simulink model "Hodgkin_Huxley"  (R2019a)
settings: Solver=VariableStepAuto  StartTime=0.0  StopTime=50  RelTol=1e-9
values from neighbouring files (symbols this model uses):
  C = 1    [H_H.m]    (also in H_H_Mod.m)
  E_k = -12    [H_H.m]    (also in H_H_Mod.m)
  E_L = 10.613    [H_H.m]    (also in H_H_Mod.m)
  E_na = 115    [H_H.m]    (also in H_H_Mod.m)
  G_k = 36    [H_H.m]    (also in H_H_Mod.m)
  G_L = 0.3    [H_H.m]    (also in H_H_Mod.m)
  G_na = 120    [H_H.m]    (also in H_H_Mod.m)
  H_init = .596    (= 0.596)    [H_H.m]    (also in H_H_Mod.m)
  I_stim = 10    [H_H.m]    (also in H_H_Mod.m = 5)
  M_init = 5.296E-2    (= 0.05296)    [H_H.m]    (also in H_H_Mod.m)
  m_pow = 5    [H_H.m]    (also in H_H_Mod.m = 3)
  N_init = 0.3177    [H_H.m]    (also in H_H_Mod.m)
  n_pow = 4    [H_H.m]    (also in H_H_Mod.m)
  t_n_gain = 3    [H_H.m]    (also in H_H_Mod.m = 1)
  T_stim_start = 10    [H_H.m]    (also in H_H_Mod.m = 1)
  T_stim_stop = 15    [H_H.m]    (also in H_H_Mod.m = 5)
  V_init = 0    [H_H.m]    (also in H_H_Mod.m)
settings Model: Creator=Pranav Maddula  LastModifiedBy=Pranav Maddula

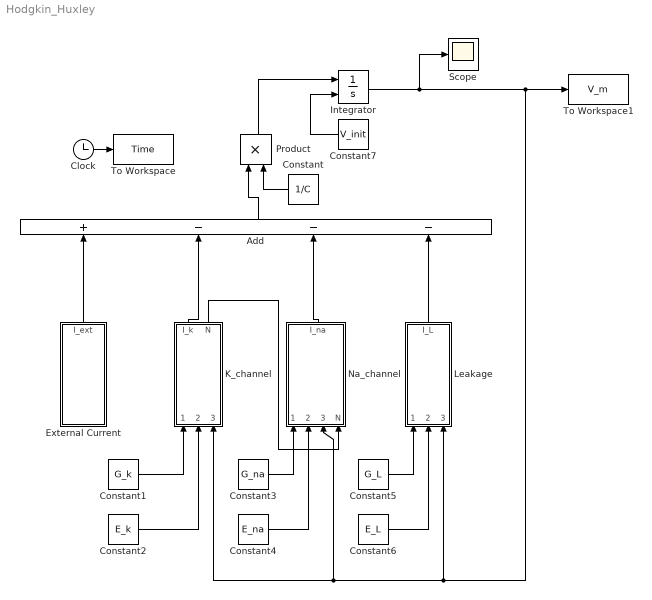
== system Hodgkin_Huxley ==
  Add : Sum  Inputs=+---
  Clock : Clock
  Constant : Constant  Value=1/C
  Constant1 : Constant  Value=G_k
  Constant2 : Constant  Value=E_k
  Constant3 : Constant  Value=G_na
  Constant4 : Constant  Value=E_na
  Constant5 : Constant  Value=G_L
  Constant6 : Constant  Value=E_L
  Constant7 : Constant  Value=V_init
  External Current : Subsystem
  Integrator : Integrator  InitialConditionSource=external
  K_channel : Subsystem
  Leakage : Subsystem
  Na_channel : Subsystem
  Product : Product
  Scope : Scope
  To Workspace : ToWorkspace  VariableName=Time  SampleTime=-1
  To Workspace1 : ToWorkspace  VariableName=V_m  SampleTime=-1
  wires:
  Clock/1 -> To Workspace/1
  External Current/1(I_ext) -> Add/1
  Leakage/1(I_L) -> Add/4
  Add/1 -> Product/1
  Constant/1 -> Product/2
  Product/1 -> Integrator/1
  Integrator/1 -> To Workspace1/1, K_channel/3(V_m), Na_channel/3(V_m), Leakage/3(V_m), Scope/1
  Constant5/1 -> Leakage/1(G_L)
  Constant6/1 -> Leakage/2(E_L)
  Constant7/1 -> Integrator/2
  K_channel/1(I_k) -> Add/2
  Na_channel/1(I_na) -> Add/3
  Constant1/1 -> K_channel/1(G_k)
  Constant2/1 -> K_channel/2(E_k)
  Constant3/1 -> Na_channel/1(G_na)
  Constant4/1 -> Na_channel/2(E_na)
  K_channel/2("N ") -> Na_channel/4(N)

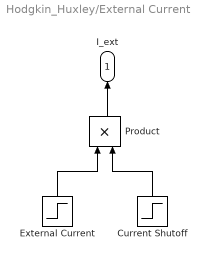
== system Hodgkin_Huxley/External Current ==
  Current Shutoff : Step  Time=T_stim_stop  Before=1  After=0  SampleTime=0
  External Current : Step  Time=T_stim_start  After=I_stim  SampleTime=0
  Product : Product
  I_ext : Outport
  wires:
  Product/1 -> I_ext/1
  External Current/1 -> Product/1
  Current Shutoff/1 -> Product/2

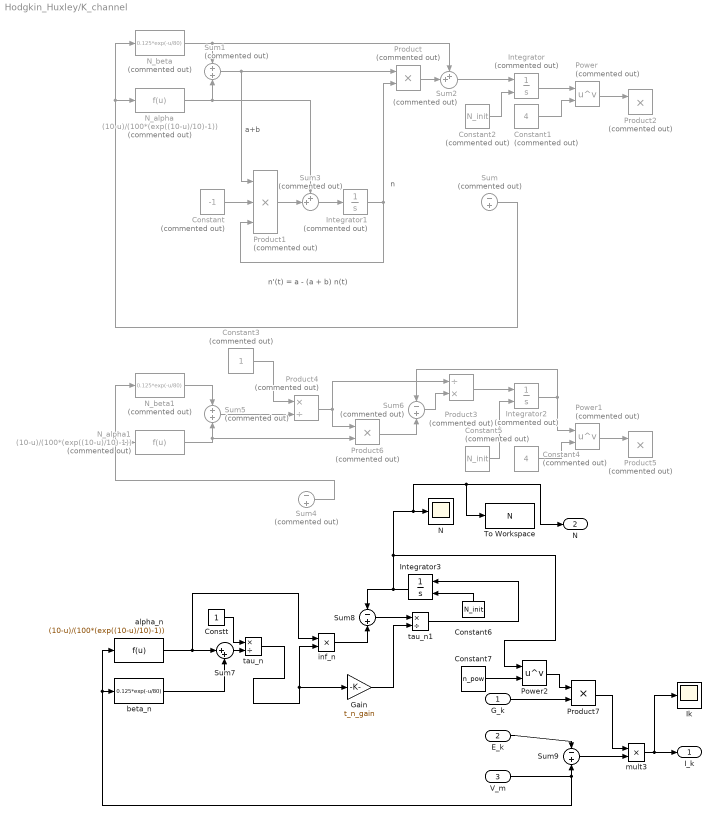
== system Hodgkin_Huxley/K_channel ==
  note: a+b
  note: n
  note: n'(t) = a - (a + b) n(t)
  G_k : Inport
  E_k : Inport  Port=2
  V_m : Inport  Port=3
  Constant : Constant  Commented=on  Value=-1
  Constant1 : Constant  Commented=on  Value=4
  Constant2 : Constant  Commented=on  Value=N_init
  Constant3 : Constant  Commented=on
  Constant4 : Constant  Commented=on  Value=4
  Constant5 : Constant  Commented=on  Value=N_init
  Constant6 : Constant  Value=N_init
  Constant7 : Constant  Value=n_pow
  Constt : Constant
  Gain : Gain  Gain=t_n_gain
  Ik : Scope
  Integrator : Integrator  Commented=on  InitialConditionSource=external
  Integrator1 : Integrator  Commented=on
  Integrator2 : Integrator  Commented=on  InitialConditionSource=external
  Integrator3 : Integrator  InitialConditionSource=external
  N : Scope
  N_alpha : Fcn  Commented=on  Expr=(10-u)/(100*(exp((10-u)/10)-1))
  N_alpha1 : Fcn  Commented=on  Expr=(10-u)/(100*(exp((10-u)/10)-1))
  N_beta : Fcn  Commented=on  Expr=0.125*exp(-u/80)
  N_beta1 : Fcn  Commented=on  Expr=0.125*exp(-u/80)
  Power : Math  Commented=on  Operator=pow  SaturateOnIntegerOverflow=on
  Power1 : Math  Commented=on  Operator=pow  SaturateOnIntegerOverflow=on
  Power2 : Math  Operator=pow  SaturateOnIntegerOverflow=on
  Product{,2,5..6} (4 alike) : Product  Commented=on
  Product1 : Product  Commented=on  Inputs=3
  Product3 : Product  Commented=on  Inputs=/*
  Product4 : Product  Commented=on  Inputs=*/
  Product7 : Product
  Sum : Sum  Commented=on  Inputs=-+
  Sum1 : Sum  Commented=on
  Sum2 : Sum  Commented=on  Inputs=++|
  Sum3 : Sum  Commented=on  Inputs=++|
  Sum4 : Sum  Commented=on  Inputs=-+
  Sum5 : Sum  Commented=on
  Sum6 : Sum  Commented=on  Inputs=-+
  Sum7 : Sum  Inputs=|++
  Sum8 : Sum  Inputs=-+
  Sum9 : Sum  Inputs=-+
  To Workspace : ToWorkspace  VariableName=N  SampleTime=-1
  alpha_n : Fcn  Expr=(10-u)/(100*(exp((10-u)/10)-1))
  beta_n : Fcn  Expr=0.125*exp(-u/80)
  inf_n : Product  Inputs=**
  mult3 : Product  Inputs=**
  tau_n : Product  Inputs=*/
  tau_n1 : Product  Inputs=*/
  I_k : Outport
  "N " : Outport  Port=2
  wires:
  N_beta/1 -> Sum2/1, Sum1/1
  N_alpha/1 -> Sum3/1, Sum1/2
  Product/1 -> Sum2/2
  Sum2/1 -> Integrator/1
  Sum1/1 -> Product1/1, Product/1
  Constant/1 -> Product1/2
  Product1/1 -> Sum3/2
  Sum3/1 -> Integrator1/1
  Integrator1/1 -> Product/2, Product1/3
  Integrator/1 -> Power/1
  Constant1/1 -> Power/2
  Power/1 -> Product2/1
  Sum/1 -> N_beta/1, N_alpha/1
  Constant2/1 -> Integrator/2
  Sum4/1 -> N_alpha1/1, N_beta1/1
  Power1/1 -> Product5/1
  N_alpha1/1 -> Product6/2, Sum5/2
  Integrator2/1 -> Power1/1, Sum6/1
  N_beta1/1 -> Sum5/1
  Constant5/1 -> Integrator2/2
  Constant4/1 -> Power1/2
  Sum5/1 -> Product4/2
  Constant3/1 -> Product4/1
  Product4/1 -> Product3/1, Product6/1
  Product6/1 -> Sum6/2
  Sum6/1 -> Product3/2
  Product3/1 -> Integrator2/1
  beta_n/1 -> Sum7/2
  alpha_n/1 -> Sum7/1, inf_n/1
  Constt/1 -> tau_n/1
  Sum8/1 -> tau_n1/1
  tau_n1/1 -> Integrator3/1
  Constant6/1 -> Integrator3/2
  Sum7/1 -> tau_n/2
  V_m/1 -> Sum9/2, beta_n/1, alpha_n/1
  Sum9/1 -> mult3/2
  E_k/1 -> Sum9/1
  G_k/1 -> Product7/2
  mult3/1 -> Ik/1, I_k/1
  inf_n/1 -> Sum8/2
  Integrator3/1 -> "N "/1, To Workspace/1, N/1, Power2/1, Sum8/1
  Constant7/1 -> Power2/2
  Power2/1 -> Product7/1
  Product7/1 -> mult3/1
  tau_n/1 -> Gain/1, inf_n/2
  Gain/1 -> tau_n1/2

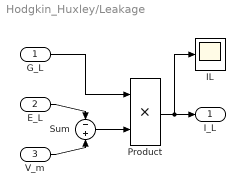
== system Hodgkin_Huxley/Leakage ==
  G_L : Inport
  E_L : Inport  Port=2
  V_m : Inport  Port=3
  IL : Scope
  Product : Product
  Sum : Sum  Inputs=-+
  I_L : Outport
  wires:
  E_L/1 -> Sum/1
  V_m/1 -> Sum/2
  Sum/1 -> Product/2
  G_L/1 -> Product/1
  Product/1 -> IL/1, I_L/1

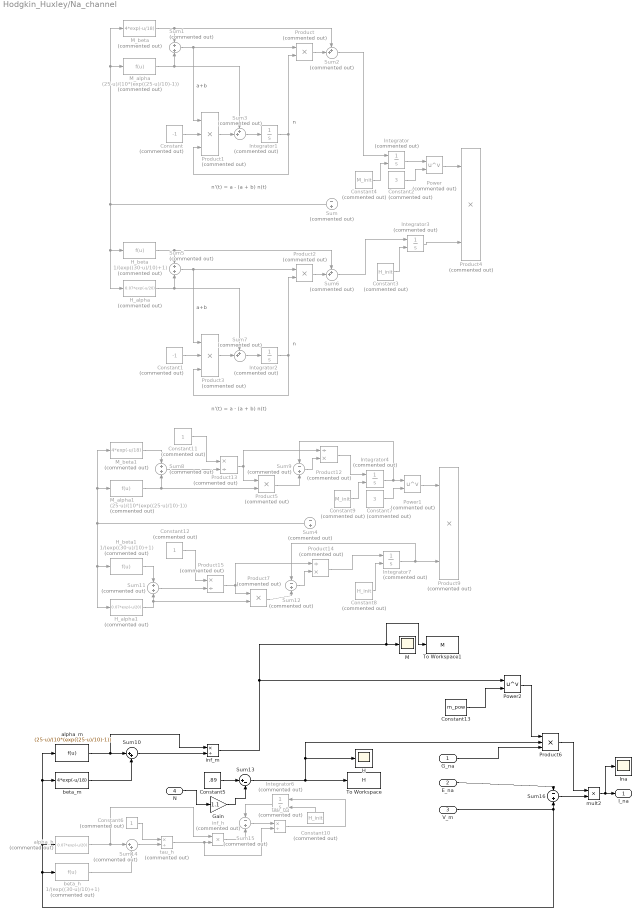
== system Hodgkin_Huxley/Na_channel ==
  note: a+b
  note: n'(t) = a - (a + b) n(t)
  note: n
  note: n'(t) = a - (a + b) n(t)
  note: a+b
  note: n
  G_na : Inport
  E_na : Inport  Port=2
  V_m : Inport  Port=3
  N : Inport  Port=4
  Constant : Constant  Commented=on  Value=-1
  Constant1 : Constant  Commented=on  Value=-1
  Constant10 : Constant  Commented=on  Value=H_init
  Constant11 : Constant  Commented=on
  Constant12 : Constant  Commented=on
  Constant13 : Constant  Value=m_pow
  Constant2 : Constant  Commented=on  Value=3
  Constant3 : Constant  Commented=on  Value=H_init
  Constant4 : Constant  Commented=on  Value=M_init
  Constant5 : Constant  Value=.89
  Constant6 : Constant  Commented=on
  Constant7 : Constant  Commented=on  Value=3
  Constant8 : Constant  Commented=on  Value=H_init
  Constant9 : Constant  Commented=on  Value=M_init
  Gain : Gain  Gain=1.1
  H : Scope
  H_alpha : Fcn  Commented=on  Expr=0.07*exp(-u/20)
  H_alpha1 : Fcn  Commented=on  Expr=0.07*exp(-u/20)
  H_beta : Fcn  Commented=on  Expr=1/(exp((30-u)/10)+1)
  H_beta1 : Fcn  Commented=on  Expr=1/(exp((30-u)/10)+1)
  Ina : Scope
  Integrator{,3..4,6..7} (5 alike) : Integrator  Commented=on  InitialConditionSource=external
  Integrator1 : Integrator  Commented=on
  Integrator2 : Integrator  Commented=on
  M : Scope
  M_alpha : Fcn  Commented=on  Expr=(25-u)/(10*(exp((25-u)/10)-1))
  M_alpha1 : Fcn  Commented=on  Expr=(25-u)/(10*(exp((25-u)/10)-1))
  M_beta : Fcn  Commented=on  Expr=4*exp(-u/18)
  M_beta1 : Fcn  Commented=on  Expr=4*exp(-u/18)
  Power : Math  Commented=on  Operator=pow  SaturateOnIntegerOverflow=on
  Power1 : Math  Commented=on  Operator=pow  SaturateOnIntegerOverflow=on
  Power2 : Math  Operator=pow  SaturateOnIntegerOverflow=on
  Product{,2,5,7} (4 alike) : Product  Commented=on
  Product{1,3..4,9} (4 alike) : Product  Commented=on  Inputs=3
  Product12 : Product  Commented=on  Inputs=/*
  Product13 : Product  Commented=on  Inputs=*/
  Product14 : Product  Commented=on  Inputs=/*
  Product15 : Product  Commented=on  Inputs=*/
  Product6 : Product  Inputs=3
  Sum{,4,9,12,15} (5 alike) : Sum  Commented=on  Inputs=-+
  Sum{1,5,8,11} (4 alike) : Sum  Commented=on
  Sum10 : Sum  Inputs=|++
  Sum13 : Sum  Inputs=|+-
  Sum14 : Sum  Commented=on  Inputs=|++
  Sum16 : Sum  Inputs=-+
  Sum{2..3,6..7} (4 alike) : Sum  Commented=on  Inputs=++|
  To Workspace : ToWorkspace  VariableName=H  SampleTime=-1
  To Workspace1 : ToWorkspace  VariableName=M  SampleTime=-1
  alpha_h : Fcn  Commented=on  Expr=0.07*exp(-u/20)
  alpha_m : Fcn  Expr=(25-u)/(10*(exp((25-u)/10)-1))
  beta_h : Fcn  Commented=on  Expr=1/(exp((30-u)/10)+1)
  beta_m : Fcn  Expr=4*exp(-u/18)
  inf_h : Product  Commented=on  Inputs=**
  inf_m : Product  Inputs=*/
  mult2 : Product  Inputs=**
  tau_h : Product  Commented=on  Inputs=*/
  tau_n5 : Product  Commented=on  Inputs=*/
  I_na : Outport
  wires:
  M_beta/1 -> Sum2/1, Sum1/1
  Sum/1 -> M_beta/1, M_alpha/1, H_alpha/1, H_beta/1
  M_alpha/1 -> Sum3/1, Sum1/2
  Sum1/1 -> Product1/1, Product/1
  Constant/1 -> Product1/2
  Sum3/1 -> Integrator1/1
  Integrator1/1 -> Product/2, Product1/3
  Product/1 -> Sum2/2
  Product1/1 -> Sum3/2
  Sum7/1 -> Integrator2/1
  Product3/1 -> Sum7/2
  Integrator2/1 -> Product2/2, Product3/3
  Product2/1 -> Sum6/2
  Constant1/1 -> Product3/2
  Sum5/1 -> Product3/1, Product2/1
  H_beta/1 -> Sum6/1, Sum5/1
  H_alpha/1 -> Sum7/1, Sum5/2
  Constant2/1 -> Power/2
  Integrator/1 -> Power/1
  Sum2/1 -> Integrator/1
  Power/1 -> Product4/1
  Integrator3/1 -> Product4/3
  Sum6/1 -> Integrator3/1
  Constant3/1 -> Integrator3/2
  Constant4/1 -> Integrator/2
  Constant8/1 -> Integrator7/2
  M_beta1/1 -> Sum8/1
  Integrator4/1 -> Sum9/1, Power1/1
  H_beta1/1 -> Sum11/1
  Power1/1 -> Product9/1
  Sum4/1 -> H_alpha1/1, H_beta1/1, M_beta1/1, M_alpha1/1
  Constant9/1 -> Integrator4/2
  Integrator7/1 -> Sum12/1, Product9/3
  Constant7/1 -> Power1/2
  Product13/1 -> Product5/1, Product12/1
  M_alpha1/1 -> Product5/2, Sum8/2
  Product5/1 -> Sum9/2
  Constant11/1 -> Product13/1
  Product12/1 -> Integrator4/1
  Sum9/1 -> Product12/2
  Sum8/1 -> Product13/2
  Product15/1 -> Product14/1, Product7/1
  H_alpha1/1 -> Product7/2, Sum11/2
  Product7/1 -> Sum12/2
  Constant12/1 -> Product15/1
  Sum12/1 -> Product14/2
  Sum11/1 -> Product15/2
  Product14/1 -> Integrator7/1
  tau_n5/1 -> Integrator6/1
  Sum16/1 -> mult2/2
  Sum14/1 -> tau_h/2
  Constant6/1 -> tau_h/1
  beta_m/1 -> Sum10/2
  beta_h/1 -> Sum14/2
  Integrator6/1 -> Sum15/1
  inf_h/1 -> Sum15/2
  E_na/1 -> Sum16/1
  Product6/1 -> mult2/1
  G_na/1 -> Product6/3
  Constant10/1 -> Integrator6/2
  alpha_m/1 -> Sum10/1, inf_m/1
  mult2/1 -> Ina/1, I_na/1
  V_m/1 -> Sum16/2, alpha_m/1, beta_m/1, alpha_h/1, beta_h/1
  Sum15/1 -> tau_n5/1
  inf_m/1 -> To Workspace1/1, M/1, Power2/1
  alpha_h/1 -> Sum14/1, inf_h/1
  tau_h/1 -> inf_h/2, tau_n5/2
  Constant13/1 -> Power2/2
  Power2/1 -> Product6/1
  Sum10/1 -> inf_m/2
  Gain/1 -> Sum13/2
  Constant5/1 -> Sum13/1
  N/1 -> Gain/1
  Sum13/1 -> Product6/2, H/1, To Workspace/1
